simulink model "validate"  (R2021a)
settings: Solver=VariableStepAuto  StartTime=0.0  StopTime=time_val  RelTol=1e-3
values from neighbouring files (symbols this model uses):
  Delta = block.DialogPrm(1).Data    [battery_dual_ekf.m]    (also in battery_dual_ekf_2.m; battery_dual_ekf_early.m; init_dekf_3.m = 0.008; kalman_validate.m)
settings Model: Creator=saleh  LastModifiedBy=saleh

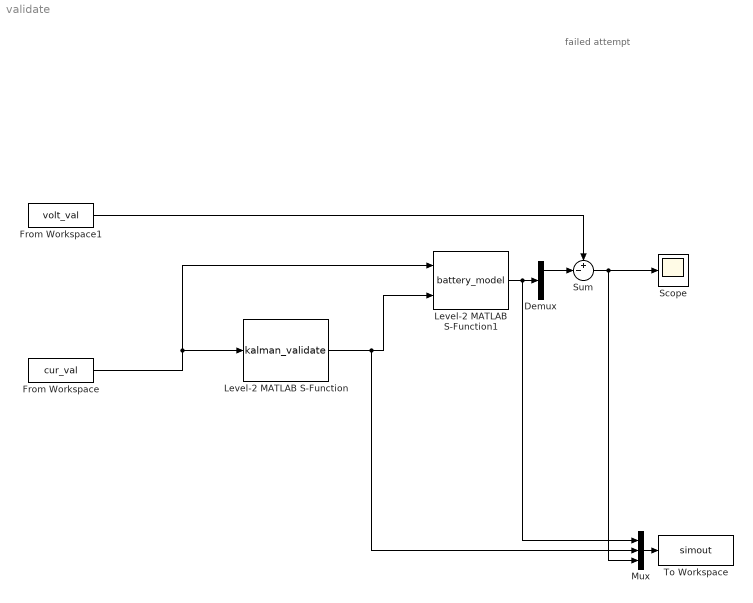
== system validate ==
  note: failed attempt
  Demux : Demux  Outputs=3
  From Workspace : FromWorkspace  VariableName=cur_val  SampleTime=Delta
  From Workspace1 : FromWorkspace  VariableName=volt_val  SampleTime=Delta
  Level-2 MATLAB S-Function : M-S-Function  FunctionName=kalman_validate  Parameters=Delta, x0, P0, a, Z_k, W_k, Qe, Cg, x_conv_2
  Level-2 MATLAB S-Function1 : M-S-Function  FunctionName=battery_model  Parameters=x_conv_2, Qe, Cg
  Mux : Mux  Inputs=3
  Scope : Scope
  Sum : Sum  Inputs=+-|
  To Workspace : ToWorkspace  VariableName=simout  SaveFormat=Timeseries  SampleTime=-1
  wires:
  From Workspace/1 -> Level-2 MATLAB S-Function1/1, Level-2 MATLAB S-Function/1
  Level-2 MATLAB S-Function/1 -> Mux/2, Level-2 MATLAB S-Function1/2
  Level-2 MATLAB S-Function1/1 -> Mux/1, Demux/1
  From Workspace1/1 -> Sum/1
  Demux/1 -> Sum/2
  Sum/1 -> Mux/3, Scope/1
  Mux/1 -> To Workspace/1
